simulink model "High_Level_Architecture_Model"  (R2025b)
settings: Solver=VariableStepAuto  StartTime=0.0  StopTime=10.0  RelTol=1e-3
settings Model: Creator=mmcda  LastModifiedBy=mmcda

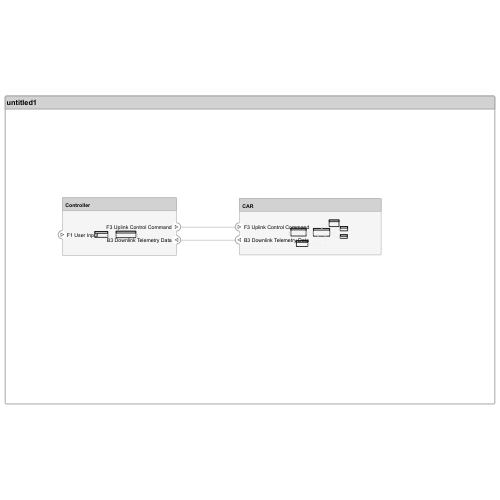
[thumbnail: Simulink's stored preview of the top-level diagram]
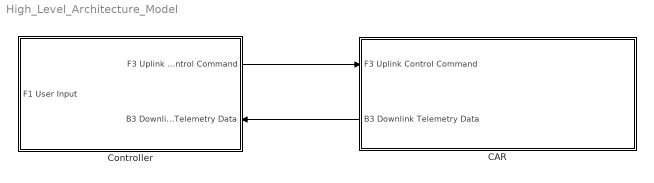
== system High_Level_Architecture_Model ==
  CAR : Subsystem
      settings: PortSchema="{\"entries\":[{\"content\":{\"headerSize\":26,\"margin\":15,\"minimumSpacing\":25,\"sides\":[{\"content\":{\"connectorIds\":[\"In1\",\"Out1\"]},\"type\":\"ConnectorPlacement.EquallySpacedRectSide\",\"uuid\":\"c98e7fb3-14a9-4f8f-8725-5d2fe99ee1e6\"},{\"content\":{\"side\":\"RIGHT\"},\"type\":\"ConnectorPlacement.EquallySpacedRectSide\",\"uuid\":\"f2023df4-7e22-4ccc-9512-d655e75621ec\"},{\"content\":{\"side\":\"TOP\"},\"type\":\"ConnectorPlacement.EquallySpacedRectSide\",\"uuid\":\"9c2c6a5d-c8f1-4d27-a6a9-5c39564f8d64\"}]},\"type\":\"ConnectorPlacement.EquallySpacedConnector\",\"uuid\":\"f2a64cbf-5e2c-4b30-b7dc-ff4495379d9a\"}],\"packageUris\":[\"http://schema.mathworks.com/mf0/Connector/R2020b\"],\"version\":\"1.0\"}"
  Controller : Subsystem
      settings: PortSchema="{\"entries\":[{\"content\":{\"headerSize\":26,\"margin\":15,\"minimumSpacing\":25,\"sides\":[{\"content\":{\"connectorIds\":[\"In2\"]},\"type\":\"ConnectorPlacement.EquallySpacedRectSide\",\"uuid\":\"c98e7fb3-14a9-4f8f-8725-5d2fe99ee1e6\"},{\"content\":{\"connectorIds\":[\"Out1\",\"In1\"],\"side\":\"RIGHT\"},\"type\":\"ConnectorPlacement.EquallySpacedRectSide\",\"uuid\":\"f2023df4-7e22-4ccc-9512-d655e75621ec\"},{\"content\":{\"side\":\"TOP\"},\"type\":\"ConnectorPlacement.EquallySpacedRectSide\",\"uuid\":\"9c2c6a5d-c8f1-4d27-a6a9-5c39564f8d64\"}]},\"type\":\"ConnectorPlacement.EquallySpacedConnector\",\"uuid\":\"f2a64cbf-5e2c-4b30-b7dc-ff4495379d9a\"}],\"packageUris\":[\"http://schema.mathworks.com/mf0/Connector/R2020b\"],\"version\":\"1.0\"}"
  wires:
  Controller/1(F3 Uplink Control Command) -> CAR/1(F3 Uplink Control Command)
  CAR/1(B3 Downlink Telemetry Data) -> Controller/1(B3 Downlink Telemetry Data)

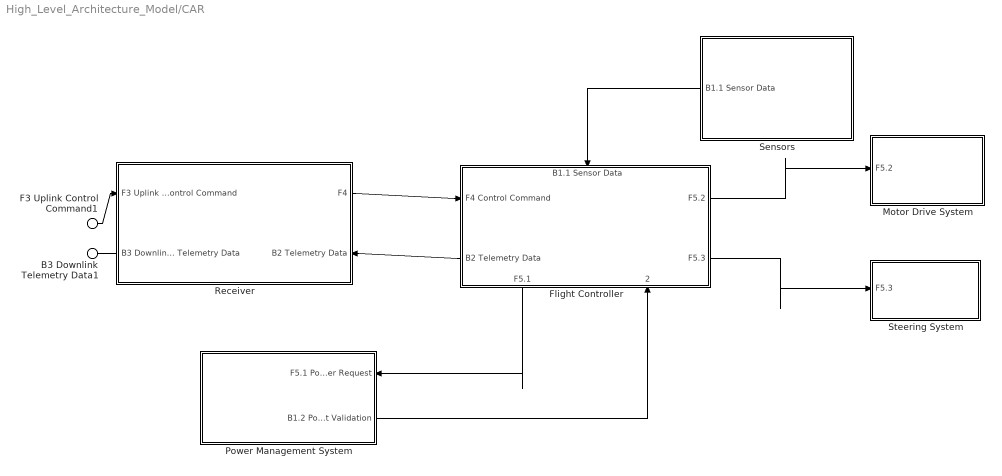
== system High_Level_Architecture_Model/CAR ==
  F3 Uplink Control Command1 : Inport  PortName=F3 Uplink Control Command
  Flight Controller : Subsystem
      settings: PortSchema="{\"entries\":[{\"content\":{\"headerSize\":26,\"margin\":15,\"minimumSpacing\":25,\"sides\":[{\"content\":{\"connectorIds\":[\"In3\",\"Out1\"]},\"type\":\"ConnectorPlacement.EquallySpacedRectSide\",\"uuid\":\"ebde801f-62a7-4f14-aaf5-010620cf3461\"},{\"content\":{\"connectorIds\":[\"Out3\",\"Out4\"],\"side\":\"RIGHT\"},\"type\":\"ConnectorPlacement.EquallySpacedRectSide\",\"uuid\":\"f0660b28-99b1-4c93-9472-8e77328b5be7\"},{\"content\":{\"connectorIds\":[\"In1\"],\"side\":\"TOP\"},\"type\":\"ConnectorPlacement.EquallySpacedRectSide\",\"uuid\":\"9672d794-05f0-4f55-b3f9-ea2756d47693\"},{\"content\":{\"connectorIds\":[\"Out2\",\"In2\"],\"side\":\"BOTTOM\"},\"type\":\"ConnectorPlacement.EquallySpacedRectSide\",\"uuid\":\"bb3a57cd-1925-49be-9ff4-2e87e1a08699\"}]},\"type\":\"ConnectorPlacement.EquallySpacedConnector\",\"uuid\":\"5f666b50-a1b1-42a3-a220-918e82a29cbf\"}],\"packageUris\":[\"http://schema.mathworks.com/mf0/Connector/R2020b\"],\"version\":\"1.0\"}"
  Motor Drive System : Subsystem
      settings: PortSchema="{\"entries\":[{\"content\":{\"headerSize\":26,\"margin\":15,\"minimumSpacing\":25,\"sides\":[{\"content\":{\"connectorIds\":[\"In1\"]},\"type\":\"ConnectorPlacement.EquallySpacedRectSide\",\"uuid\":\"ebde801f-62a7-4f14-aaf5-010620cf3461\"},{\"content\":{\"side\":\"RIGHT\"},\"type\":\"ConnectorPlacement.EquallySpacedRectSide\",\"uuid\":\"f0660b28-99b1-4c93-9472-8e77328b5be7\"},{\"content\":{\"side\":\"TOP\"},\"type\":\"ConnectorPlacement.EquallySpacedRectSide\",\"uuid\":\"9672d794-05f0-4f55-b3f9-ea2756d47693\"},{\"content\":{\"side\":\"BOTTOM\"},\"type\":\"ConnectorPlacement.EquallySpacedRectSide\",\"uuid\":\"3028ae02-f403-49d7-bc0b-14d36f54ea7c\"}]},\"type\":\"ConnectorPlacement.EquallySpacedConnector\",\"uuid\":\"5f666b50-a1b1-42a3-a220-918e82a29cbf\"}],\"packageUris\":[\"http://schema.mathworks.com/mf0/Connector/R2020b\"],\"version\":\"1.0\"}"
  Power Management System : Subsystem
      settings: PortSchema="{\"entries\":[{\"content\":{\"headerSize\":26,\"margin\":15,\"minimumSpacing\":25,\"sides\":[{\"content\":{},\"type\":\"ConnectorPlacement.EquallySpacedRectSide\",\"uuid\":\"ebde801f-62a7-4f14-aaf5-010620cf3461\"},{\"content\":{\"connectorIds\":[\"In1\",\"Out1\"],\"side\":\"RIGHT\"},\"type\":\"ConnectorPlacement.EquallySpacedRectSide\",\"uuid\":\"f0660b28-99b1-4c93-9472-8e77328b5be7\"},{\"content\":{\"side\":\"TOP\"},\"type\":\"ConnectorPlacement.EquallySpacedRectSide\",\"uuid\":\"9672d794-05f0-4f55-b3f9-ea2756d47693\"}]},\"type\":\"ConnectorPlacement.EquallySpacedConnector\",\"uuid\":\"5f666b50-a1b1-42a3-a220-918e82a29cbf\"}],\"packageUris\":[\"http://schema.mathworks.com/mf0/Connector/R2020b\"],\"version\":\"1.0\"}"
  Receiver : Subsystem
      settings: PortSchema="{\"entries\":[{\"content\":{\"headerSize\":26,\"margin\":15,\"minimumSpacing\":25,\"sides\":[{\"content\":{\"connectorIds\":[\"In2\",\"Out2\"]},\"type\":\"ConnectorPlacement.EquallySpacedRectSide\",\"uuid\":\"ebde801f-62a7-4f14-aaf5-010620cf3461\"},{\"content\":{\"connectorIds\":[\"Out1\",\"In1\"],\"side\":\"RIGHT\"},\"type\":\"ConnectorPlacement.EquallySpacedRectSide\",\"uuid\":\"f0660b28-99b1-4c93-9472-8e77328b5be7\"},{\"content\":{\"side\":\"TOP\"},\"type\":\"ConnectorPlacement.EquallySpacedRectSide\",\"uuid\":\"9672d794-05f0-4f55-b3f9-ea2756d47693\"}]},\"type\":\"ConnectorPlacement.EquallySpacedConnector\",\"uuid\":\"5f666b50-a1b1-42a3-a220-918e82a29cbf\"}],\"packageUris\":[\"http://schema.mathworks.com/mf0/Connector/R2020b\"],\"version\":\"1.0\"}"
  Sensors : Subsystem
      settings: PortSchema="{\"entries\":[{\"content\":{\"headerSize\":26,\"margin\":15,\"minimumSpacing\":25,\"sides\":[{\"content\":{\"connectorIds\":[\"Out1\"]},\"type\":\"ConnectorPlacement.EquallySpacedRectSide\",\"uuid\":\"ebde801f-62a7-4f14-aaf5-010620cf3461\"},{\"content\":{\"side\":\"RIGHT\"},\"type\":\"ConnectorPlacement.EquallySpacedRectSide\",\"uuid\":\"f0660b28-99b1-4c93-9472-8e77328b5be7\"},{\"content\":{\"side\":\"TOP\"},\"type\":\"ConnectorPlacement.EquallySpacedRectSide\",\"uuid\":\"9672d794-05f0-4f55-b3f9-ea2756d47693\"}]},\"type\":\"ConnectorPlacement.EquallySpacedConnector\",\"uuid\":\"5f666b50-a1b1-42a3-a220-918e82a29cbf\"}],\"packageUris\":[\"http://schema.mathworks.com/mf0/Connector/R2020b\"],\"version\":\"1.0\"}"
  Steering System : Subsystem
      settings: PortSchema="{\"entries\":[{\"content\":{\"headerSize\":26,\"margin\":15,\"minimumSpacing\":25,\"sides\":[{\"content\":{\"connectorIds\":[\"In1\"]},\"type\":\"ConnectorPlacement.EquallySpacedRectSide\",\"uuid\":\"ebde801f-62a7-4f14-aaf5-010620cf3461\"},{\"content\":{\"side\":\"RIGHT\"},\"type\":\"ConnectorPlacement.EquallySpacedRectSide\",\"uuid\":\"f0660b28-99b1-4c93-9472-8e77328b5be7\"},{\"content\":{\"side\":\"TOP\"},\"type\":\"ConnectorPlacement.EquallySpacedRectSide\",\"uuid\":\"9672d794-05f0-4f55-b3f9-ea2756d47693\"}]},\"type\":\"ConnectorPlacement.EquallySpacedConnector\",\"uuid\":\"5f666b50-a1b1-42a3-a220-918e82a29cbf\"}],\"packageUris\":[\"http://schema.mathworks.com/mf0/Connector/R2020b\"],\"version\":\"1.0\"}"
  B3 Downlink Telemetry Data1 : Outport  PortName=B3 Downlink Telemetry Data
  wires:
  Receiver/2(B3 Downlink Telemetry Data) -> B3 Downlink Telemetry Data1/1
  Flight Controller/1(B2 Telemetry Data) -> Receiver/1(B2 Telemetry Data)
  Flight Controller/2(F5.1) -> Power Management System/1("F5.1 Power Request ")
  Flight Controller/3(F5.2) -> Motor Drive System/1(F5.2)
  Power Management System/1(B1.2 Power Request Validation) -> Flight Controller/2(B1.2 Power Request Validation)
  F3 Uplink Control Command1/1 -> Receiver/2("F3 Uplink Control Command ")
  Receiver/1(F4) -> Flight Controller/3(F4 Control Command)
  Flight Controller/4(F5.3) -> Steering System/1(F5.3)
  Sensors/1(B1.1 Sensor Data) -> Flight Controller/1(B1.1 Sensor Data)

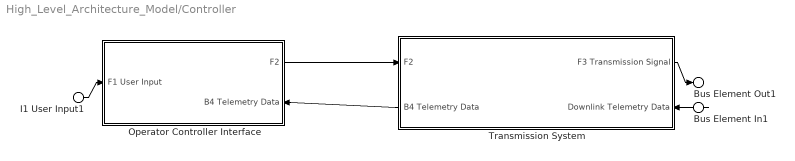
== system High_Level_Architecture_Model/Controller ==
  Bus Element In1 : Inport  PortName=B3 Downlink Telemetry Data
  I1 User Input1 : Inport  Port=2  PortName=F1 User Input
  Operator Controller Interface : Subsystem
      settings: PortSchema="{\"entries\":[{\"content\":{\"headerSize\":26,\"margin\":15,\"minimumSpacing\":25,\"sides\":[{\"content\":{\"connectorIds\":[\"In2\"]},\"type\":\"ConnectorPlacement.EquallySpacedRectSide\",\"uuid\":\"ebde801f-62a7-4f14-aaf5-010620cf3461\"},{\"content\":{\"connectorIds\":[\"Out1\",\"In1\"],\"side\":\"RIGHT\"},\"type\":\"ConnectorPlacement.EquallySpacedRectSide\",\"uuid\":\"f0660b28-99b1-4c93-9472-8e77328b5be7\"},{\"content\":{\"side\":\"TOP\"},\"type\":\"ConnectorPlacement.EquallySpacedRectSide\",\"uuid\":\"9672d794-05f0-4f55-b3f9-ea2756d47693\"}]},\"type\":\"ConnectorPlacement.EquallySpacedConnector\",\"uuid\":\"5f666b50-a1b1-42a3-a220-918e82a29cbf\"}],\"packageUris\":[\"http://schema.mathworks.com/mf0/Connector/R2020b\"],\"version\":\"1.0\"}"
  Transmission System : Subsystem
      settings: PortSchema="{\"entries\":[{\"content\":{\"headerSize\":26,\"margin\":15,\"minimumSpacing\":25,\"sides\":[{\"content\":{\"connectorIds\":[\"In2\",\"Out1\"]},\"type\":\"ConnectorPlacement.EquallySpacedRectSide\",\"uuid\":\"ebde801f-62a7-4f14-aaf5-010620cf3461\"},{\"content\":{\"connectorIds\":[\"Out2\",\"In1\"],\"side\":\"RIGHT\"},\"type\":\"ConnectorPlacement.EquallySpacedRectSide\",\"uuid\":\"f0660b28-99b1-4c93-9472-8e77328b5be7\"},{\"content\":{\"side\":\"TOP\"},\"type\":\"ConnectorPlacement.EquallySpacedRectSide\",\"uuid\":\"9672d794-05f0-4f55-b3f9-ea2756d47693\"}]},\"type\":\"ConnectorPlacement.EquallySpacedConnector\",\"uuid\":\"5f666b50-a1b1-42a3-a220-918e82a29cbf\"}],\"packageUris\":[\"http://schema.mathworks.com/mf0/Connector/R2020b\"],\"version\":\"1.0\"}"
  Bus Element Out1 : Outport  PortName=F3 Uplink Control Command
  wires:
  Operator Controller Interface/1(F2) -> Transmission System/2(F2)
  I1 User Input1/1 -> Operator Controller Interface/2(F1 User Input)
  Transmission System/2(F3 Transmission Signal) -> Bus Element Out1/1
  Bus Element In1/1 -> Transmission System/1(Downlink Telemetry Data)
  Transmission System/1(B4 Telemetry Data) -> Operator Controller Interface/1(B4 Telemetry Data)

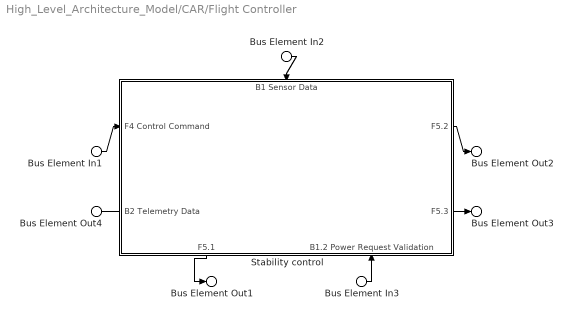
== system High_Level_Architecture_Model/CAR/Flight Controller ==
  Bus Element In2 : Inport  PortName=B1.1 Sensor Data
  Bus Element In3 : Inport  Port=2  PortName=B1.2 Power Request Validation
  Bus Element In1 : Inport  Port=3  PortName=F4 Control Command
  "Stability control " : Subsystem
      settings: PortSchema="{\"entries\":[{\"content\":{\"headerSize\":26,\"margin\":15,\"minimumSpacing\":25,\"sides\":[{\"content\":{\"connectorIds\":[\"In3\",\"Out4\"]},\"type\":\"ConnectorPlacement.EquallySpacedRectSide\",\"uuid\":\"ebde801f-62a7-4f14-aaf5-010620cf3461\"},{\"content\":{\"connectorIds\":[\"Out2\",\"Out3\"],\"side\":\"RIGHT\"},\"type\":\"ConnectorPlacement.EquallySpacedRectSide\",\"uuid\":\"f0660b28-99b1-4c93-9472-8e77328b5be7\"},{\"content\":{\"connectorIds\":[\"In1\"],\"side\":\"TOP\"},\"type\":\"ConnectorPlacement.EquallySpacedRectSide\",\"uuid\":\"9672d794-05f0-4f55-b3f9-ea2756d47693\"},{\"content\":{\"connectorIds\":[\"Out1\",\"In2\"],\"side\":\"BOTTOM\"},\"type\":\"ConnectorPlacement.EquallySpacedRectSide\",\"uuid\":\"3621ed21-7a26-47e7-9ca9-08af29ee204a\"}]},\"type\":\"ConnectorPlacement.EquallySpacedConnector\",\"uuid\":\"5f666b50-a1b1-42a3-a220-918e82a29cbf\"}],\"packageUris\":[\"http://schema.mathworks.com/mf0/Connector/R2020b\"],\"version\":\"1.0\"}"
  Bus Element Out4 : Outport  PortName=B2 Telemetry Data
  Bus Element Out1 : Outport  Port=2  PortName=F5.1
  Bus Element Out2 : Outport  Port=3  PortName=F5.2
  Bus Element Out3 : Outport  Port=4  PortName=F5.3
  wires:
  Bus Element In1/1 -> "Stability control "/3(F4 Control Command)
  "Stability control "/4(B2 Telemetry Data) -> Bus Element Out4/1
  Bus Element In2/1 -> "Stability control "/1(B1 Sensor Data)
  Bus Element In3/1 -> "Stability control "/2(B1.2 Power Request Validation)
  "Stability control "/2(F5.2) -> Bus Element Out2/1
  "Stability control "/3(F5.3) -> Bus Element Out3/1
  "Stability control "/1(F5.1) -> Bus Element Out1/1

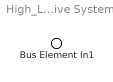
== system High_Level_Architecture_Model/CAR/Motor Drive System ==
  Bus Element In1 : Inport  PortName=F5.2

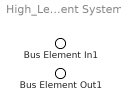
== system High_Level_Architecture_Model/CAR/Power Management System ==
  Bus Element In1 : Inport  PortName=F5.1 Power Request
  Bus Element Out1 : Outport  PortName=B1.2 Power Request Validation

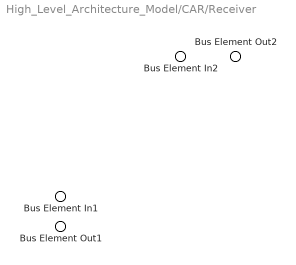
== system High_Level_Architecture_Model/CAR/Receiver ==
  Bus Element In2 : Inport  PortName=B2 Telemetry Data
  Bus Element In1 : Inport  Port=2  PortName=F3 Uplink Control Command
  Bus Element Out2 : Outport  PortName=F4
  Bus Element Out1 : Outport  Port=2  PortName=B3 Downlink Telemetry Data

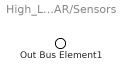
== system High_Level_Architecture_Model/CAR/Sensors ==
  Out Bus Element1 : Outport  PortName=B1.1 Sensor Data

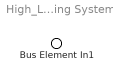
== system High_Level_Architecture_Model/CAR/Steering System ==
  Bus Element In1 : Inport  PortName=F5.3

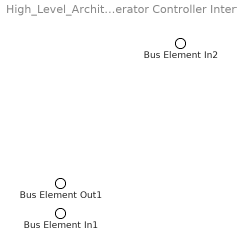
== system High_Level_Architecture_Model/Controller/Operator Controller Interface ==
  Bus Element In2 : Inport  PortName=B4 Telemetry Data
  Bus Element In1 : Inport  Port=2  PortName=F1 User Input
  Bus Element Out1 : Outport  PortName=F2

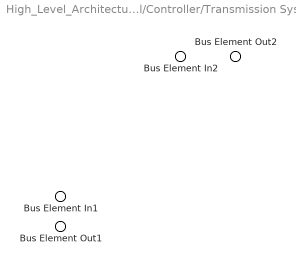
== system High_Level_Architecture_Model/Controller/Transmission System ==
  Bus Element In2 : Inport  PortName=Downlink Telemetry Data
  Bus Element In1 : Inport  Port=2  PortName=F2
  Bus Element Out2 : Outport  PortName=B4 Telemetry Data
  Bus Element Out1 : Outport  Port=2  PortName=F3 Transmission Signal

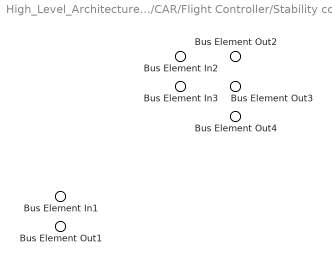
== system High_Level_Architecture_Model/CAR/Flight Controller/Stability control  ==
  Bus Element In2 : Inport  PortName=B1 Sensor Data
  Bus Element In3 : Inport  Port=2  PortName=B1.2 Power Request Validation
  Bus Element In1 : Inport  Port=3  PortName=F4 Control Command
  Bus Element Out4 : Outport  PortName=F5.1
  Bus Element Out2 : Outport  Port=2  PortName=F5.2
  Bus Element Out3 : Outport  Port=3  PortName=F5.3
  Bus Element Out1 : Outport  Port=4  PortName=B2 Telemetry Data
